simulink library "aerolib3dof2"  (Simulink 5.0)
values from neighbouring files (symbols this model uses):
  s = aeroliblist    [asbhelp.m]
undefined symbols (not defined in the file or in its folder): m
libraries: aerolib3dof2 x2, aerolib3dofsys x1, aerolibutil x1, aerolibtransform2 x1, aerolibconvert x1
settings Model: Creator=sgage  LastModifiedBy=sgage  ExtModeAutoUpdateStatusClock=off

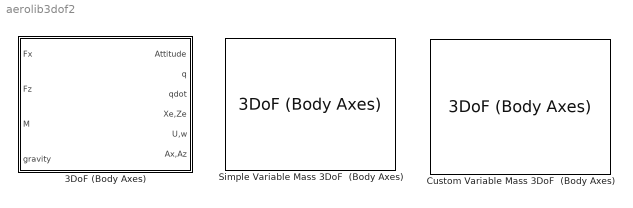
== system aerolib3dof2 ==
  3DoF (Body Axes) : Subsystem  mask(3DoF EoM){units=Metric (MKS), mtype=Fixed, v_ini=100, theta_ini=0, alpha_ini=0, q_ini=0, pos_ini=[0 0], mass=1.0, mass_e=0.5, mass_f=3.0, Iyy=1.0, Iyy_e=0.5, Iyy_f=3.0, g_in=External, g=9.81}
      mask prompts: mtype "Mass type:"; v_ini "Initial velocity:"; theta_ini "Initial body attitude:"; alpha_ini "Initial incidence:"; q_ini "Initial body rotation rate:"; pos_ini "Initial position (x z):"; mass "Initial mass:"; mass_e "Empty mass:"; mass_f "Full mass:"; Iyy "Inertia:"; Iyy_e "Empty inertia:"; Iyy_f "Full inertia:"; g_in "Gravity source:"; g "Acceleration due to gravity:"
      mask help: Integrate the three-degrees-of-freedom equations of motion to determine body position, velocity, attitude, and related values.
      mask init:
      | U0 = v_ini*cos(alpha_ini);
      | w0 = v_ini*sin(alpha_ini);
      | [x y xp yp highstr lowstr maxy miny]=aeroimage('threedofbody');
      | ports=aeroicon('aeroblk3dofbody','icon');
      mask Help: web(asbhelp('3dofbodyaxes'));
      mask StyleString: popup(Metric (MKS)|English (Velocity in ft/s)|English (Velocity in kts)),popup(Fixed|Simple Variable|Custom Variable),edit,edit,edit,edit,edit,edit,edit,edit,edit,edit,edit,popup(Internal|External),edit
      mask CallbackString: aeroicon('aeroblk3dofbody');|aeroicon('aeroblk3dofbody');||||||||||||aeroicon('aeroblk3dofbody');|
      mask Display:
      | port_label(ports(1).type,ports(1).port,ports(1).txt,'texmode','on');
      | port_label(ports(2).type,ports(2).port,ports(2).txt,'texmode','on');
      | port_label(ports(3).type,ports(3).port,ports(3).txt,'texmode','on');
      | port_label(ports(4).type,ports(4).port,ports(4).txt,'texmode','on');
      | port_label(ports(5).type,ports(5).port,ports(5).txt,'texmode','on');
      | port_label(ports(6).type,ports(6).port,ports(6).txt,'texmode','on');
      | port_label(ports(7).type,ports(7).port,ports(7).txt,'texmode','on');
      | port_label(ports(8).type,ports(8).port,ports(8).txt,'texmode','on');
      | port_label(ports(9).type,ports(9).port,ports(9).txt,'texmode','on');
      | port_label(ports(10).type,ports(10).port,ports(10).txt,'texmode','on');
      | port_label(ports(11).type,ports(11).port,ports(11).txt,'texmode','on');
      | port_label(ports(12).type,ports(12).port,ports(12).txt,'texmode','on');
      | port_label(ports(13).type,ports(13).port,ports(13).txt,'texmode','on');
      | port_label(ports(14).type,ports(14).port,ports(14).txt,'texmode','on');
      | port_label(ports(15).type,ports(15).port,ports(15).txt,'texmode','on');
      | plot(x,y);
      | patch(xp, yp);
      | text(0.5,maxy+0.05,highstr{:},'horizontalAlignment','center')
      | text(0.5,miny-0.05,lowstr{:},'horizontalAlignment','center')
  Custom Variable Mass 3DoF  (Body Axes) : aerolib3dof2/3DoF (Body Axes)  units=Metric (MKS)  mtype=Custom Variable  v_ini=100  theta_ini=0  alpha_ini=0  q_ini=0  pos_ini=[0 0]  mass=1.0  mass_e=0.5  mass_f=3.0  Iyy=1.0  Iyy_e=0.5  Iyy_f=3.0  g_in=External  g=9.81
  Simple Variable Mass 3DoF  (Body Axes) : aerolib3dof2/3DoF (Body Axes)  units=Metric (MKS)  mtype=Simple Variable  v_ini=100  theta_ini=0  alpha_ini=0  q_ini=0  pos_ini=[0 0]  mass=1.0  mass_e=0.5  mass_f=3.0  Iyy=1.0  Iyy_e=0.5  Iyy_f=3.0  g_in=External  g=9.81

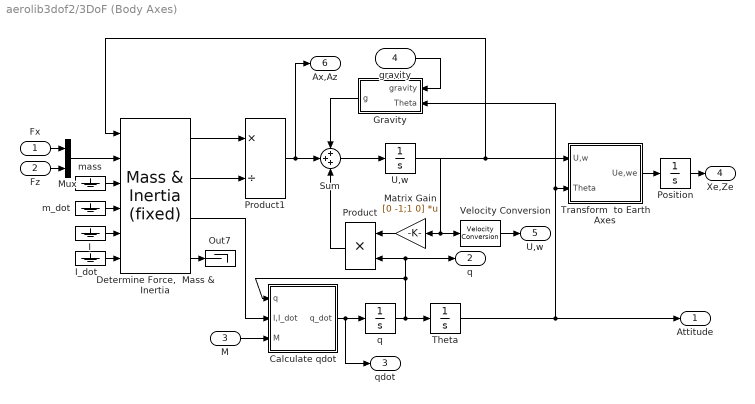
== system aerolib3dof2/3DoF (Body Axes) ==
  Fx : Inport
  Fz : Inport  Port=2
  M : Inport  Port=3
  gravity : Inport  Port=4
  Calculate qdot : Subsystem
  "Determine Force,  Mass & Inertia" : aerolib3dofsys/Mass & Inertia (fixed)
  Gravity : Subsystem  Orientation=left
  I : Ground
  I_dot : Ground
  Matrix Gain : Gain  Orientation=left  Gain=[0 -1;1 0]  Multiplication=Matrix(K*u)  SaturateOnIntegerOverflow=on
  Mux : Mux  Inputs=2
  Out7 : Terminator
  Position : Integrator  InitialCondition=pos_ini
  Product : Product  Orientation=left  SaturateOnIntegerOverflow=on  InputSameDT=on
  Product1 : Product  Inputs=*/  SaturateOnIntegerOverflow=on
  Sum : Sum  Inputs=+++  SaturateOnIntegerOverflow=on
  Theta : Integrator  InitialCondition=theta_ini
  Transform  to Earth Axes : Subsystem
  U,w : Integrator  InitialCondition=[U0 w0]
  Velocity Conversion : aerolibconvert/Velocity Conversion  IU=m/s  OU=m/s
  m_dot : Ground
  mass : Ground
  q : Integrator  InitialCondition=q_ini
  Attitude : Outport  InitialOutput=0
  "q " : Outport  Port=2  InitialOutput=0
  qdot : Outport  Port=3  InitialOutput=0
  Xe,Ze : Outport  Port=4  InitialOutput=0
  "U,w  " : Outport  Port=5  InitialOutput=0
  Ax,Az : Outport  Port=6  InitialOutput=0
  wires:
  Gravity/1(g) -> Sum/1
  Product1/1 -> Ax,Az/1, Sum/2
  Product/1 -> Sum/3
  Mux/1 -> "Determine Force,  Mass & Inertia"/2
  Fz/1 -> Mux/2
  Fx/1 -> Mux/1
  Transform  to Earth Axes/1(Ue,we) -> Position/1
  Matrix Gain/1 -> Product/1
  Position/1 -> Xe,Ze/1
  U,w/1 -> Transform  to Earth Axes/1(U,w), "Determine Force,  Mass & Inertia"/1, Matrix Gain/1, Velocity Conversion/1
  Theta/1 -> Transform  to Earth Axes/2(Theta), Gravity/2(Theta), Attitude/1
  Calculate qdot/1(q_dot) -> qdot/1, q/1
  M/1 -> Calculate qdot/3(M)
  q/1 -> Theta/1, Product/2, "q "/1, Calculate qdot/1(q)
  Sum/1 -> U,w/1
  "Determine Force,  Mass & Inertia"/2 -> Product1/2
  "Determine Force,  Mass & Inertia"/1 -> Product1/1
  "Determine Force,  Mass & Inertia"/3 -> Calculate qdot/2(I,I_dot)
  mass/1 -> "Determine Force,  Mass & Inertia"/3
  m_dot/1 -> "Determine Force,  Mass & Inertia"/4
  I/1 -> "Determine Force,  Mass & Inertia"/5
  I_dot/1 -> "Determine Force,  Mass & Inertia"/6
  gravity/1 -> Gravity/1(gravity)
  "Determine Force,  Mass & Inertia"/4 -> Out7/1
  Velocity Conversion/1 -> "U,w  "/1

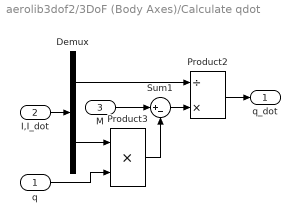
== system aerolib3dof2/3DoF (Body Axes)/Calculate qdot ==
  q : Inport
  I,I_dot : Inport  Port=2
  M : Inport  Port=3
  Demux : Demux  Outputs=2
  Product2 : Product  Inputs=/*  SaturateOnIntegerOverflow=on  InputSameDT=on
  Product3 : Product  SaturateOnIntegerOverflow=on  InputSameDT=on
  Sum1 : Sum  Inputs=|+-  SaturateOnIntegerOverflow=on
  q_dot : Outport
  wires:
  Sum1/1 -> Product2/2
  Product3/1 -> Sum1/2
  q/1 -> Product3/2
  Product2/1 -> q_dot/1
  M/1 -> Sum1/1
  Demux/2 -> Product3/1
  Demux/1 -> Product2/1
  I,I_dot/1 -> Demux/1

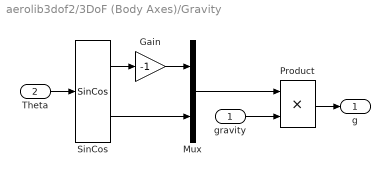
== system aerolib3dof2/3DoF (Body Axes)/Gravity ==
  gravity : Inport
  Theta : Inport  Port=2
  Gain : Gain  Gain=-1  SaturateOnIntegerOverflow=on
  Mux : Mux  Inputs=2
  Product : Product  SaturateOnIntegerOverflow=on  InputSameDT=on
  SinCos : aerolibutil/SinCos
  g : Outport
  wires:
  gravity/1 -> Product/2
  Product/1 -> g/1
  Mux/1 -> Product/1
  SinCos/2 -> Mux/2
  Gain/1 -> Mux/1
  SinCos/1 -> Gain/1
  Theta/1 -> SinCos/1

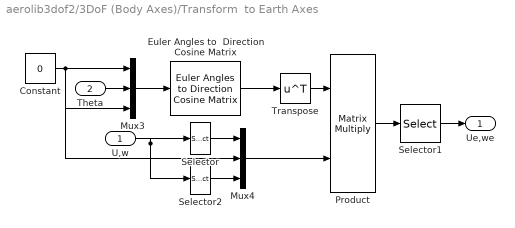
== system aerolib3dof2/3DoF (Body Axes)/Transform  to Earth Axes ==
  U,w : Inport
  Theta : Inport  Port=2
  Constant : Constant  Value=0
  Euler Angles to  Direction Cosine Matrix : aerolibtransform2/Euler Angles to  Direction Cosine Matrix
  Mux3 : Mux  Inputs=3
  Mux4 : Mux  Inputs=3
  Product : Product  Multiplication=Matrix(*)  SaturateOnIntegerOverflow=on
  Selector : Selector  InputPortWidth=2
  Selector1 : Selector  Elements=[1 3]  InputPortWidth=3
  Selector2 : Selector  Elements=2  InputPortWidth=2
  Transpose : Math  Operator=transpose
  Ue,we : Outport
  wires:
  Transpose/1 -> Product/1
  Theta/1 -> Mux3/2
  U,w/1 -> Selector/1, Selector2/1
  Mux3/1 -> Euler Angles to  Direction Cosine Matrix/1
  Constant/1 -> Mux3/1, Mux3/3, Mux4/2
  Euler Angles to  Direction Cosine Matrix/1 -> Transpose/1
  Mux4/1 -> Product/2
  Product/1 -> Selector1/1
  Selector1/1 -> Ue,we/1
  Selector/1 -> Mux4/1
  Selector2/1 -> Mux4/3
